simulink model "MBD_GoTo_From"  (R2021b)
settings: Solver=FixedStepDiscrete  StartTime=0.0  StopTime=10.0  FixedStep=0.01  RelTol=1e-3
settings Model: Creator=waleed.elshemy  LastModifiedBy=waleed.elshemy

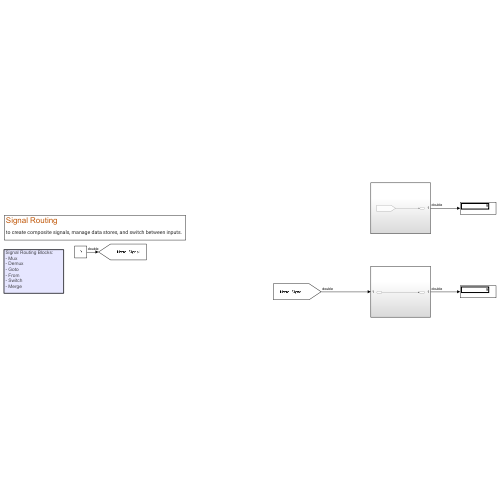
[thumbnail: Simulink's stored preview of the top-level diagram]
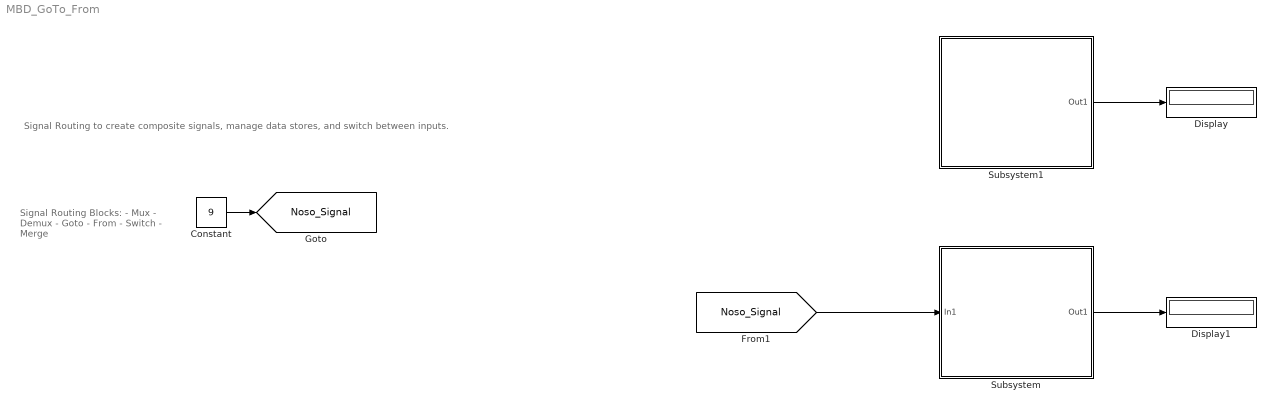
== system MBD_GoTo_From ==
  note: Signal Routing
      | to create composite signals, manage data stores, and switch between inputs.
  note: Signal Routing Blocks:
      | - Mux
      | - Demux
      | - Goto
      | - From
      | - Switch
      | - Merge
  Constant : Constant  Value=9
  Display : Display
  Display1 : Display
  Subsystem : Subsystem
  Subsystem1 : Subsystem
  tag scope: Noso_Signal=global
  wires:
  Constant/1 -> [Noso_Signal]
  [Noso_Signal] -> Subsystem/1(In1)
  Subsystem1/1(Out1) -> Display/1
  Subsystem/1(Out1) -> Display1/1

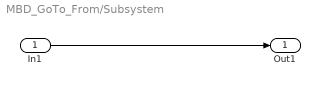
== system MBD_GoTo_From/Subsystem ==
  In1 : Inport
  Out1 : Outport
  wires:
  In1/1 -> Out1/1

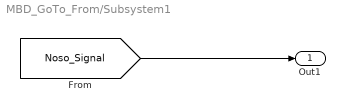
== system MBD_GoTo_From/Subsystem1 ==
  Out1 : Outport
  wires:
  [Noso_Signal] -> Out1/1
